simulink model "AbstractFuelControl_M1_FP"  (R2013a)
settings: Solver=ode15s  SolverMode=SingleTasking  StartTime=0  StopTime=simTime  FixedStep=1e-04  RelTol=1e-06  AbsTol=1e-06
values from neighbouring files (symbols this model uses):
  AF_sensor_tol = 1.0    (= 1)    [AbstractFuelControl.m]    (also in AbstractFuelControl_BB.m; AbstractFuelControl_FR.m)
  fault_time = 60    [AbstractFuelControl.m]    (also in AbstractFuelControl_BB.m; AbstractFuelControl_FR.m)
  fuel_inj_tol = 1.0    (= 1)    [AbstractFuelControl.m]    (also in AbstractFuelControl_BB.m; AbstractFuelControl_FR.m)
  MAF_sensor_tol = 1.0    (= 1)    [AbstractFuelControl.m]    (also in AbstractFuelControl_BB.m; AbstractFuelControl_FR.m)
  measureTime = 1    [AbstractFuelControl.m]    (also in AbstractFuelControl_BB.m; AbstractFuelControl_FR.m)
  simTime = 50    [AbstractFuelControl.m]    (also in AbstractFuelControl_BB.m = 15; AbstractFuelControl_FR.m = 12)
  spec_num = 1    [AbstractFuelControl.m]    (also in AbstractFuelControl_BB.m; AbstractFuelControl_FR.m)
(part 2 of 2)

== system AbstractFuelControl_M1_FP/Model 1/AF_Controller/fuel_controller/fuel_controller_10ms/air_estimation/down_scale12 ==
  In1 : Inport
  Constant8 : Constant  Value=100000  OutDataTypeStr=Inherit: Inherit via back propagation  SampleTime=-1
      settings: AttributesFormatString=Value = %<Value>
  Divide2 : Product  Inputs=*/  OutDataTypeStr=Inherit: Inherit via back propagation
  Out1 : Outport
  wires:
  Constant8/1 -> Divide2/2
  Divide2/1 -> Out1/1
  In1/1 -> Divide2/1

== system AbstractFuelControl_M1_FP/Model 1/AF_Controller/fuel_controller/fuel_controller_10ms/air_estimation/down_scale13 ==
  In1 : Inport
  Constant8 : Constant  Value=100  OutDataTypeStr=Inherit: Inherit via back propagation  SampleTime=-1
      settings: AttributesFormatString=Value = %<Value>
  Divide2 : Product  Inputs=*/  OutDataTypeStr=Inherit: Inherit via back propagation
  Out1 : Outport
  wires:
  Constant8/1 -> Divide2/2
  Divide2/1 -> Out1/1
  In1/1 -> Divide2/1

== system AbstractFuelControl_M1_FP/Model 1/AF_Controller/fuel_controller/fuel_controller_10ms/air_estimation/down_scale14 ==
  In1 : Inport
  Constant8 : Constant  Value=10  OutDataTypeStr=Inherit: Inherit via back propagation  SampleTime=-1
      settings: AttributesFormatString=Value = %<Value>
  Divide2 : Product  Inputs=*/  OutDataTypeStr=Inherit: Inherit via back propagation
  Out1 : Outport
  wires:
  Constant8/1 -> Divide2/2
  Divide2/1 -> Out1/1
  In1/1 -> Divide2/1

== system AbstractFuelControl_M1_FP/Model 1/AF_Controller/fuel_controller/fuel_controller_10ms/air_estimation/down_scale2 ==
  In1 : Inport
  Constant8 : Constant  Value=10  OutDataTypeStr=Inherit: Inherit via back propagation  SampleTime=-1
      settings: AttributesFormatString=Value = %<Value>
  Divide2 : Product  Inputs=*/  OutDataTypeStr=Inherit: Inherit via back propagation
  Out1 : Outport
  wires:
  Constant8/1 -> Divide2/2
  Divide2/1 -> Out1/1
  In1/1 -> Divide2/1

== system AbstractFuelControl_M1_FP/Model 1/AF_Controller/fuel_controller/fuel_controller_10ms/air_estimation/down_scale3 ==
  In1 : Inport
  Constant8 : Constant  Value=10000  OutDataTypeStr=Inherit: Inherit via back propagation  SampleTime=-1
      settings: AttributesFormatString=Value = %<Value>
  Divide2 : Product  Inputs=*/  OutDataTypeStr=Inherit: Inherit via back propagation
  Out1 : Outport
  wires:
  Constant8/1 -> Divide2/2
  Divide2/1 -> Out1/1
  In1/1 -> Divide2/1

== system AbstractFuelControl_M1_FP/Model 1/AF_Controller/fuel_controller/fuel_controller_10ms/air_estimation/down_scale4 ==
  In1 : Inport
  Constant8 : Constant  Value=10  OutDataTypeStr=Inherit: Inherit via back propagation  SampleTime=-1
      settings: AttributesFormatString=Value = %<Value>
  Divide2 : Product  Inputs=*/  OutDataTypeStr=Inherit: Inherit via back propagation
  Out1 : Outport
  wires:
  Constant8/1 -> Divide2/2
  Divide2/1 -> Out1/1
  In1/1 -> Divide2/1

== system AbstractFuelControl_M1_FP/Model 1/AF_Controller/fuel_controller/fuel_controller_10ms/air_estimation/down_scale5 ==
  In1 : Inport
  Constant8 : Constant  Value=100  OutDataTypeStr=Inherit: Inherit via back propagation  SampleTime=-1
      settings: AttributesFormatString=Value = %<Value>
  Divide2 : Product  Inputs=*/  OutDataTypeStr=Inherit: Inherit via back propagation
  Out1 : Outport
  wires:
  Constant8/1 -> Divide2/2
  Divide2/1 -> Out1/1
  In1/1 -> Divide2/1

== system AbstractFuelControl_M1_FP/Model 1/AF_Controller/fuel_controller/fuel_controller_10ms/air_estimation/down_scale7 ==
  In1 : Inport
  Constant8 : Constant  Value=100  OutDataTypeStr=Inherit: Inherit via back propagation  SampleTime=-1
      settings: AttributesFormatString=Value = %<Value>
  Divide2 : Product  Inputs=*/  OutDataTypeStr=Inherit: Inherit via back propagation
  Out1 : Outport
  wires:
  Constant8/1 -> Divide2/2
  Divide2/1 -> Out1/1
  In1/1 -> Divide2/1

== system AbstractFuelControl_M1_FP/Model 1/AF_Controller/fuel_controller/fuel_controller_10ms/air_estimation/down_scale9 ==
  In1 : Inport
  Constant8 : Constant  Value=10  OutDataTypeStr=Inherit: Inherit via back propagation  SampleTime=-1
      settings: AttributesFormatString=Value = %<Value>
  Divide2 : Product  Inputs=*/  OutDataTypeStr=Inherit: Inherit via back propagation
  Out1 : Outport
  wires:
  Constant8/1 -> Divide2/2
  Divide2/1 -> Out1/1
  In1/1 -> Divide2/1

== system AbstractFuelControl_M1_FP/Model 1/AF_Controller/fuel_controller/fuel_controller_10ms/feedback_PI_controller/down_scale1 ==
  In1 : Inport
  Constant8 : Constant  OutDataTypeStr=Inherit: Inherit via back propagation  SampleTime=-1
      settings: AttributesFormatString=Value = %<Value>
  Divide2 : Product  Inputs=*/  OutDataTypeStr=Inherit: Inherit via back propagation
  Out1 : Outport
  wires:
  Constant8/1 -> Divide2/2
  Divide2/1 -> Out1/1
  In1/1 -> Divide2/1

== system AbstractFuelControl_M1_FP/Model 1/AF_Controller/fuel_controller/fuel_controller_10ms/feedback_PI_controller/down_scale2 ==
  In1 : Inport
  Constant8 : Constant  Value=1000  OutDataTypeStr=Inherit: Inherit via back propagation  SampleTime=-1
      settings: AttributesFormatString=Value = %<Value>
  Divide2 : Product  Inputs=*/  OutDataTypeStr=Inherit: Inherit via back propagation
  Out1 : Outport
  wires:
  Constant8/1 -> Divide2/2
  Divide2/1 -> Out1/1
  In1/1 -> Divide2/1
